simulink model "Problem6_15_BlockDiagram"  (R2020b)
settings: Solver=VariableStepAuto  StartTime=0.0  StopTime=500  RelTol=1e-3
values from neighbouring files (symbols this model uses):
  G_den = cell2mat(G_den)    [Problem6_15.m]
  G_num = cell2mat(G_num)    [Problem6_15.m]
  K_den = cell2mat(K_den)    [Problem6_15.m]
  K_num = cell2mat(K_num)    [Problem6_15.m]
  Kp = 10    [Problem6_14.m]    (also in Problem6_15.m; Problem6_8.m = 1)
  t_final = 500    [Problem6_15.m]
settings Model: Creator=jonathanmoran  LastModifiedBy=jonathanmoran

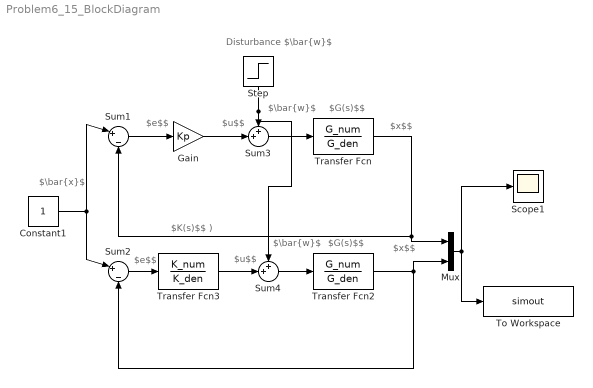
== system Problem6_15_BlockDiagram ==
  note: $x$$
  note: $\bar{x}$
  note: $e$$
  note: $u$$
  note: $K(s)$$ )
  note: $G(s)$$
  note: Disturbance $\bar{w}$
  note: $\bar{w}$
  note: $G(s)$$
  note: $e$$
  note: $u$$
  note: $\bar{w}$
  note: $x$$
  Constant1 : Constant  SampleTime=t_final
  Gain : Gain  Gain=Kp
  Mux : Mux  Inputs=2
  Scope1 : Scope
  Step : Step  After=10  SampleTime=t_final
  Sum1 : Sum  Inputs=|+|-
  Sum2 : Sum  Inputs=|+|-
  Sum3 : Sum  Inputs=++|
  Sum4 : Sum  Inputs=++|
  To Workspace : ToWorkspace  VariableName=simout  SampleTime=-1
  Transfer Fcn : TransferFcn  Numerator=G_num  Denominator=G_den
  Transfer Fcn2 : TransferFcn  Numerator=G_num  Denominator=G_den
  Transfer Fcn3 : TransferFcn  Numerator=K_num  Denominator=K_den
  wires:
  Mux/1 -> Scope1/1, To Workspace/1
  Sum2/1 -> Transfer Fcn3/1
  Transfer Fcn/1 -> Sum1/2, Mux/1
  Transfer Fcn2/1 -> Mux/2, Sum2/2
  Sum3/1 -> Transfer Fcn/1
  Gain/1 -> Sum3/2
  Step/1 -> Sum4/1, Sum3/1
  Sum1/1 -> Gain/1
  Sum4/1 -> Transfer Fcn2/1
  Transfer Fcn3/1 -> Sum4/2
  Constant1/1 -> Sum1/1, Sum2/1
